simulink subsystem "Write_ULOG_Disabled"  (R2025a)
settings: Solver=VariableStepAuto  StartTime=0.0  StopTime=10.0  RelTol=1e-3
settings Model: Creator=gurt1  LastModifiedBy=gurt1
settings RTWCC: GPUComputeCapability=3.5

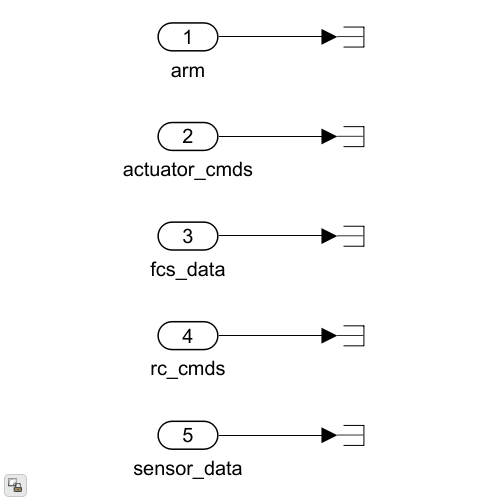
[thumbnail: Simulink's stored preview of the top-level diagram]
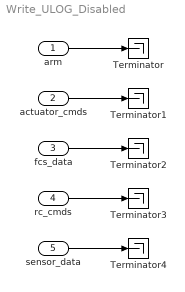
== system Write_ULOG_Disabled ==
  arm : Inport
  actuator_cmds : Inport  Port=2
  fcs_data : Inport  Port=3
  rc_cmds : Inport  Port=4
  sensor_data : Inport  Port=5
  Terminator{,1..4} (5 alike) : Terminator
  wires:
  fcs_data/1 -> Terminator2/1
  actuator_cmds/1 -> Terminator1/1
  arm/1 -> Terminator/1
  rc_cmds/1 -> Terminator3/1
  sensor_data/1 -> Terminator4/1
